simulink model "simu_t3"  (R2024a)
settings: Solver=VariableStepAuto  StartTime=0.0  StopTime=10.0  RelTol=1e-3
undefined symbols (not defined in the file): A, B, C, D, h_rastreio, k1_rastreio, k1_reg, k2_rastreio, k2_reg
libraries: dspsrcs4 x1
settings Model: Creator=carlo  LastModifiedBy=carlo

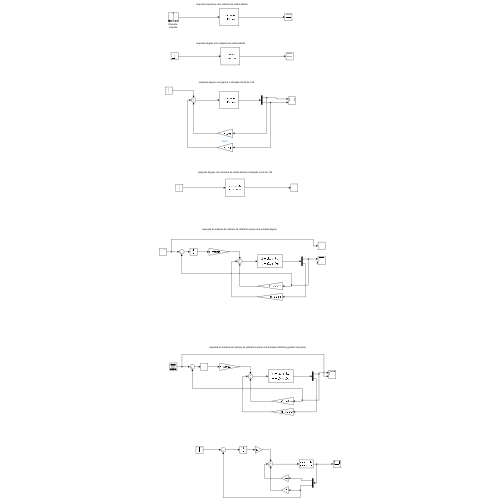
[thumbnail: Simulink's stored preview of the top-level diagram]
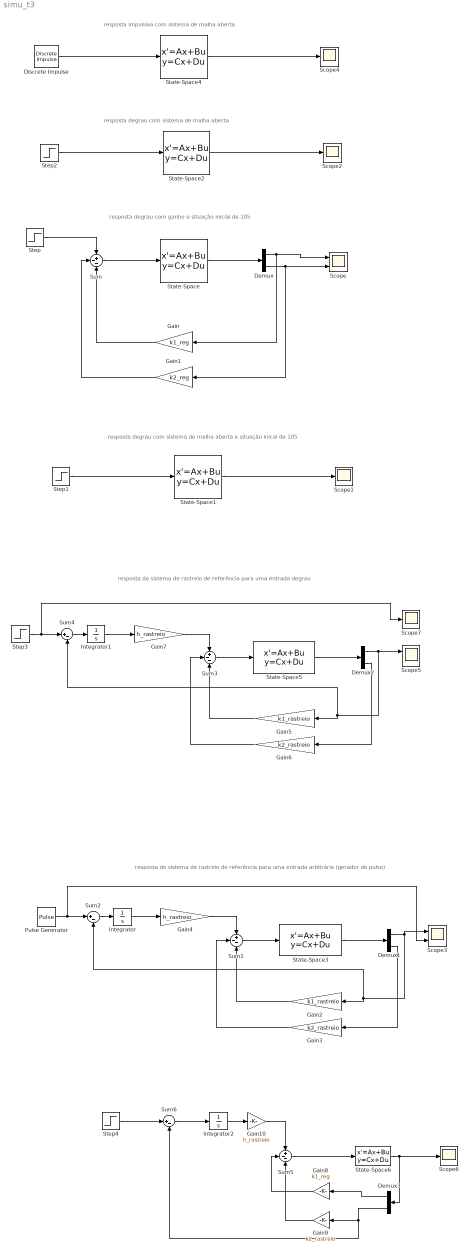
== system simu_t3 ==
  note: resposta impulsiva com sistema de malha aberta
  note: resposta do sistema de rastreio de referência para uma entrada arbitrária (gerador de pulso)
  note: resposta degrau com sistema de malha aberta
  note: resposta degrau com ganho e situação inicial de 105
  note: resposta degrau com sistema de malha aberta e situação inical de 105
  note: resposta do sistema de rastreio de referência para uma entrada degrau
  Demux{,1..3} (4 alike) : Demux  Outputs=2
  Discrete Impulse : dspsrcs4/Discrete  Impulse  Delay=0  SampleTime=1  FrameSample=1  OutputFrames=off  dataType=double  isSigned=on  wordLen=16  udDataType=sfix(16)  fracBitsMode=Best precision  numFracBits=15  OutDataTypeStr=double  LastOutDataTypeStr=double
  Gain : Gain  Gain=k1_reg
  Gain1 : Gain  Gain=k2_reg
  Gain10 : Gain  Gain=h_rastreio
  Gain2 : Gain  Gain=k1_rastreio
  Gain3 : Gain  Gain=k2_rastreio
  Gain4 : Gain  Gain=h_rastreio
  Gain5 : Gain  Gain=k1_rastreio
  Gain6 : Gain  Gain=k2_rastreio
  Gain7 : Gain  Gain=h_rastreio
  Gain8 : Gain  Gain=k1_reg
  Gain9 : Gain  Gain=k2_rastreio
  Integrator : Integrator
  Integrator1 : Integrator
  Integrator2 : Integrator
  Pulse Generator : DiscretePulseGenerator  Amplitude=50  Period=10  PulseWidth=5  SampleTime=0.4
  Scope : Scope  NumInputPorts=2
  Scope{1..2,4,6..7} (5 alike) : Scope
  Scope3 : Scope  NumInputPorts=2
  Scope5 : Scope  NumInputPorts=2
  State-Space{,2..5} (5 alike) : StateSpace  A=A  B=B  C=C  D=D  InitialCondition=0
  State-Space1 : StateSpace  A=A  B=B  C=C  D=D  InitialCondition=[105 0]
  State-Space6 : StateSpace  A=A  B=B  C=C  D=D  InitialCondition=[0 ;0]
  Step{,1..4} (5 alike) : Step  SampleTime=0
  Sum{,1,3,5} (4 alike) : Sum  Inputs=+--
  Sum2 : Sum  Inputs=|+-
  Sum4 : Sum  Inputs=|+-
  Sum6 : Sum  Inputs=|+-
  wires:
  Demux/2 -> Gain1/1, Scope/2
  Demux/1 -> Gain/1, Scope/1
  State-Space/1 -> Demux/1
  Sum/1 -> State-Space/1
  Gain/1 -> Sum/3
  Gain1/1 -> Sum/2
  Step/1 -> Sum/1
  Step1/1 -> State-Space1/1
  State-Space1/1 -> Scope1/1
  State-Space2/1 -> Scope2/1
  Step2/1 -> State-Space2/1
  State-Space3/1 -> Demux1/1
  Pulse Generator/1 -> Scope3/2, Sum2/1
  Integrator/1 -> Gain4/1
  Demux1/1 -> Sum2/2, Gain2/1, Scope3/1
  Gain2/1 -> Sum1/3
  Sum1/1 -> State-Space3/1
  Sum2/1 -> Integrator/1
  Gain4/1 -> Sum1/1
  Gain3/1 -> Sum1/2
  Demux1/2 -> Gain3/1
  State-Space4/1 -> Scope4/1
  Discrete Impulse/1 -> State-Space4/1
  Demux2/2 -> Gain6/1
  Gain6/1 -> Sum3/2
  Gain7/1 -> Sum3/1
  Sum4/1 -> Integrator1/1
  Sum3/1 -> State-Space5/1
  Gain5/1 -> Sum3/3
  Demux2/1 -> Scope5/1, Gain5/1, Sum4/2
  Integrator1/1 -> Gain7/1
  Step3/1 -> Scope7/1, Sum4/1
  State-Space5/1 -> Demux2/1
  Gain10/1 -> Sum5/1
  Sum6/1 -> Integrator2/1
  Gain9/1 -> Sum5/3
  Step4/1 -> Sum6/1
  Integrator2/1 -> Gain10/1
  State-Space6/1 -> Demux3/1, Scope6/1
  Demux3/2 -> Gain9/1, Sum6/2
  Gain8/1 -> Sum5/2
  Demux3/1 -> Gain8/1
  Sum5/1 -> State-Space6/1
